simulink model "scara_robot_model"  (R2025b)
settings: Solver=VariableStepAuto  StartTime=0.0  StopTime=10  RelTol=1e-3
model workspace: external: MATLAB File C:\Users\Mehdi\Documents\Phase3\Model\SOLIDWORK_PR3_MehdiSadeghian_Model_DataFile1.m (data not in the file)
undefined symbols (not defined in the file or in its folder): smiData, X, Y, Z
libraries: sm_lib x27, nesl_utility x24, slpidlib x4
(part 2 of 2)

== matlab function scara_robot_model/Trajectory Generator ==
  data: t input; tf input; q1_actual input; q2_actual input; d4_actual input; X_target input; q1_d output; q2_d output; Y_target input; Z_target input; L1 input; L2 input; q3_d output; d4_d output
function [q1_d, q2_d, q3_d, d4_d] = Trajectory_Generator(t, tf, q1_actual, q2_actual, d4_actual, X_target, Y_target, Z_target, L1, L2)    
    persistent X_start Y_start Z_start
    
    if isempty(X_start)
        X_start = L1 * cos(q1_actual) + L2 * cos(q1_actual + q2_actual);
        Z_start = L1 * sin(q1_actual) + L2 * sin(q1_actual + q2_actual);
        Y_start = d4_actual;
    end
    
    tau = min(t, tf) / tf;
    if tf > 0
        s = 10*(tau^3) - 15*(tau^4) + 6*(tau^5);
    else
        s = 1;
    end
    
    xd = X_start + (X_target - X_start) * s;
    yd = Y_start + (Y_target - Y_start) * s;
    zd = Z_start + (Z_target - Z_start) * s;
    
    if (xd^2 + zd^2) > (L1 + L2)^2
        warning('Target out of reach');
    end
    
    % Inverse Kinematics
    c2 = (xd^2 + zd^2 - L1^2 - L2^2) / (2 * L1 * L2);

    c2 = max(-1, min(1, c2)); 
    s2 = sqrt(1 - c2^2); 
    
    q2_d = atan2(s2, c2);
    q1_d = atan2(zd, xd) - atan2(L2*s2, L1 + L2*c2);
    
    
    q3_d = 0;
    d4_d = yd;
    
end
